simulink model "IIRFilter"  (R2023a)
settings: Solver=VariableStepAuto  StartTime=0.0  StopTime=2*48/fs  RelTol=1e-3
values from neighbouring files (symbols this model uses):
  a = [a0 a1 a2]    [band_pass_filter.m]    (also in high_pass_filter.m; low_pass_filter.m; peak_filter.m; peak_filter1.m = [a0 a1 a2]/a0)
  b = [b0 b1 b2]    [band_pass_filter.m]    (also in high_pass_filter.m; low_pass_filter.m; peak_filter.m; peak_filter1.m = [b0 b1 b2]/a0)
  fs = 48e3    (= 48000)    [dibujarHz.m]    (also in test_script.m)
settings Model: Creator=pausa  LastModifiedBy=pausa

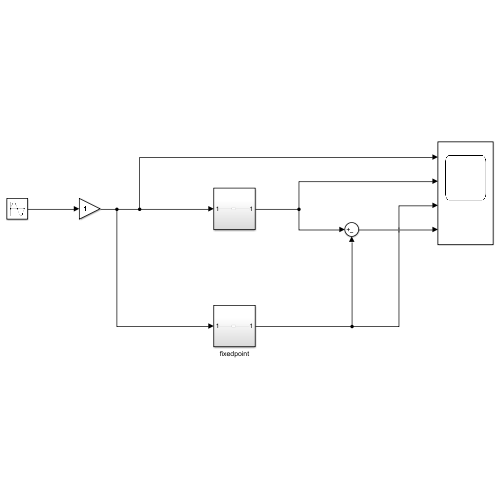
[thumbnail: Simulink's stored preview of the top-level diagram]
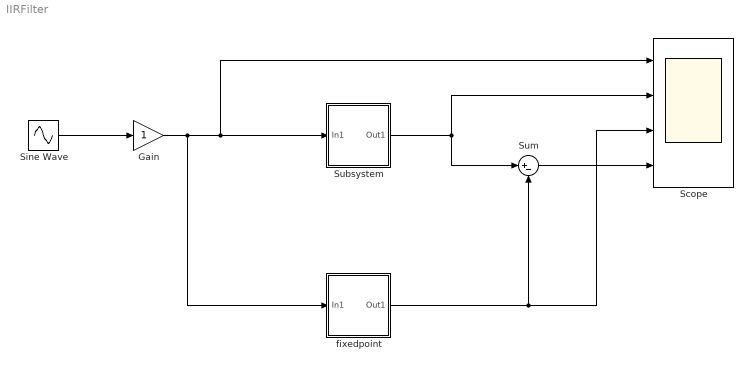
== system IIRFilter ==
  Gain : Gain  OutDataTypeStr=fixdt(1,24,23)  LockScale=on
  Scope : Scope  NumInputPorts=4
  Sine Wave : Sin  SineType=Sample based  Amplitude=0.3  Samples=60  SampleTime=1/fs
  Subsystem : Subsystem
  Sum : Sum  Inputs=|+-
  fixedpoint : Subsystem
  wires:
  Sine Wave/1 -> Gain/1
  Subsystem/1(Out1) -> Scope/2, Sum/1
  fixedpoint/1(Out1) -> Scope/3, Sum/2
  Sum/1 -> Scope/4
  Gain/1 -> fixedpoint/1(In1), Scope/1, Subsystem/1(In1)

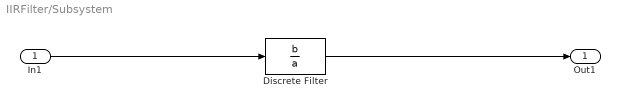
== system IIRFilter/Subsystem ==
  In1 : Inport
  Discrete Filter : DiscreteFilter  Numerator=b  Denominator=a  FilterStructure=Direct form I  NumCoefDataTypeStr=fixdt(1,18,16)  DenCoefDataTypeStr=fixdt(1,18,16)  OutDataTypeStr=Inherit: Same as input
  Out1 : Outport
  wires:
  Discrete Filter/1 -> Out1/1
  In1/1 -> Discrete Filter/1

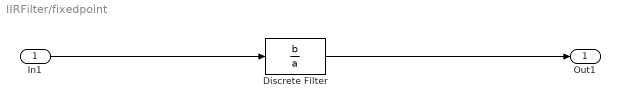
== system IIRFilter/fixedpoint ==
  In1 : Inport
  Discrete Filter : DiscreteFilter  Numerator=b  Denominator=a  FilterStructure=Direct form I  NumCoefDataTypeStr=fixdt(1,18,16)  DenCoefDataTypeStr=fixdt(1,18,16)  NumProductDataTypeStr=fixdt(1,42,39)  DenProductDataTypeStr=fixdt(1,42,39)  NumAccumDataTypeStr=fixdt(1,44,39)  DenAccumDataTypeStr=fixdt(1,44,39)  OutDataTypeStr=fixdt(1,24,23)
  Out1 : Outport
  wires:
  In1/1 -> Discrete Filter/1
  Discrete Filter/1 -> Out1/1
